simulink model "ObjectDetectLabConditions"  (R2019a)
settings: Solver=FixedStepAuto  StartTime=0.0  StopTime=inf  RelTol=1e-3  EnableMultiTasking=on
undefined symbols (not defined in the file): strel
libraries: embdlinuxlib x5, visionstatistics x1, visiontextngfix x1, visionmorphops x1
settings Model: SimulationMode=external  Creator=Shilpa  LastModifiedBy=Shilpa
settings SolverCC: PositivePriorityOrder=on
settings DataIOCC: ReturnWorkspaceOutputs=off
settings OptimizationCC: PassReuseOutputArgsAs=Individual arguments  MaxStackSize=64
settings DebuggingCC: ParameterTunabilityLossMsg=error  ArithmeticOperatorsInVariantConditions=warning
settings HardwareCC: ProdBitPerPointer=32  ProdBitPerSizeT=32  ProdBitPerPtrDiffT=32  ProdLargestAtomicInteger=Long  ProdLargestAtomicFloat=Double  ProdWordSize=32  ProdHWDeviceType=ARM Compatible->ARM Cortex
settings ModelReferenceCC: UpdateModelReferenceTargets=Force
settings SFSimCC: SimUseLocalCustomCode=off  MATLABDynamicMemAlloc=off
settings RTWCC: SystemTargetFile=ert.tlc  HardwareBoard=Raspberry Pi  TLCOptions="-aInlineSetEventsForThisBaseRateFcn=TLC_FALSE -aSuppressMultiTaskScheduler=TLC_FALSE  -aRateBasedStepFcn=0"  TemplateMakefile=ert_default_tmf  GenerateReport=on  RTWUseLocalCustomCode=off  Toolchain=GNU GCC Raspberry Pi  IncludeHyperlinkInReport=on  LaunchReport=on  GenerateTraceInfo=on  GenerateTraceReport=on  GenerateTraceReportSl=on  GenerateTraceReportSf=on  GenerateTraceReportEml=on
settings CodeAppCC: ForceParamTrailComments=on  IgnoreCustomStorageClasses=off  OperatorAnnotations=on  SimulinkDataObjDesc=on  SFDataObjDesc=on  MATLABFcnDesc=on  InsertBlockDesc=on  StateflowObjectComments=on  MATLABSourceComments=on
settings ERTTargetCC: SupportVariableSizeSignals=on

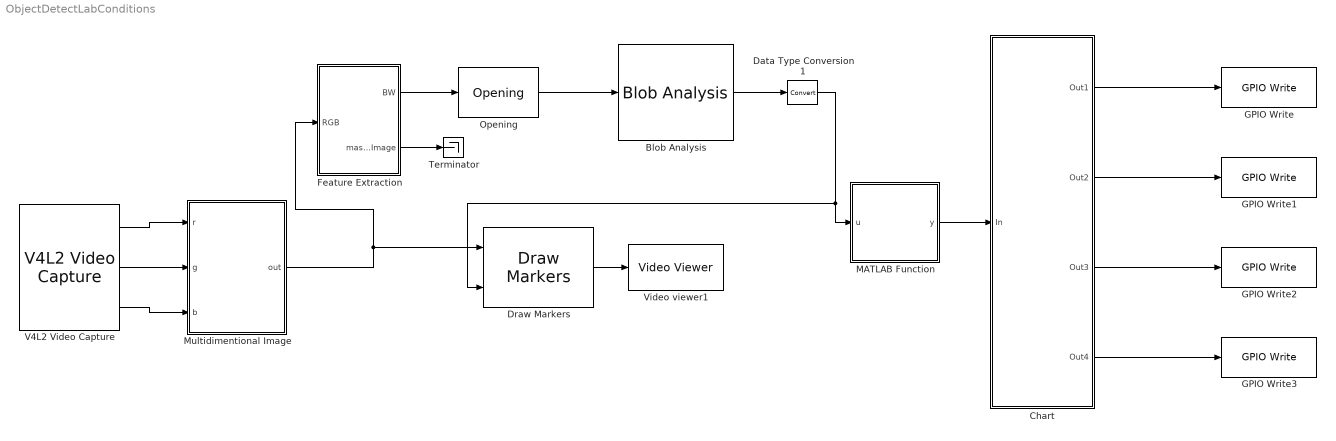
== system ObjectDetectLabConditions ==
  Blob Analysis : visionstatistics/Blob Analysis  Tag=vipblks_row_conv  area=off  centroid=on  bBox=off  majorAxis=off  minorAxis=off  angle=off  eccentricity=off  equivDiameterSq=off  extent=off  perimeter=off  outDT=double  conn=8  isLabel=off  maxBlobs=50  warnIfNumBlobsExceeded=on  isCount=off  useMinArea=off  minArea=0  useMaxArea=off  maxArea=intmax('uint32')  excludeBorderBlob=off  isOutVarDim=off  isFill=on  fillValues=-1  roundingMode=Floor  overflowMode=off  prodOutputMode=Binary point scaling  prodOutputWordLength=32  prodOutputFracLength=16  prodOutputSlope=2^-16  accumMode=Binary point scaling  accumWordLength=32  accumFracLength=0  accumSlope=2^0  outputMode=Binary point scaling  outputWordLength=32  outputFracLength=16  outputSlope=2^-16  memorySlope=2^-16  firstCoeffMode=Binary point scaling  firstCoeffWordLength=16  firstCoeffFracLength=14  firstCoeffSlope=2^-14  secondCoeffMode=Binary point scaling  secondCoeffWordLength=32  secondCoeffFracLength=16  secondCoeffSlope=2^-16
      settings: SourceProductName=Computer Vision Toolbox
  Chart : Stateflow chart  TreatAsAtomicUnit=on
  Data Type Conversion1 : DataTypeConversion
  Draw Markers : visiontextngfix/Draw Markers  shape=X-mark  size=4  fill=off  fillClrSource=Specify via dialog  display=White  intensity=200  color=[200 255 100]  opacity=0.6  viewport=Entire image  antialiasing=off  inType=Obsolete  imagePorts=One multidimensional signal  roundingMode=Floor  overflowMode=off  memoryMode=Specify word length  memoryWordLength=16  memoryFracLength=15  memorySlope=2^-14  prodOutputMode=Binary point scaling  prodOutputWordLength=32  prodOutputFracLength=14  prodOutputSlope=2^-14  accumSlope=2^-14
      settings: SourceProductName=Computer Vision Toolbox  SourceProductBaseCode=VP
  Feature Extraction : MATLAB Function  TreatAsAtomicUnit=on
  GPIO Write : embdlinuxlib/GPIO Write  board=Pi 2 Model B  gpio=23  direction=Output  blockPlatform=Raspberry Pi
      settings: SourceProductName=Simulink Coder Support Package for BeagleBone Blue Hardware  SourceProductBaseCode=SC_BEAGLEBONE_BLUE
  GPIO Write1 : embdlinuxlib/GPIO Write  board=Pi 2 Model B  gpio=24  direction=Output  blockPlatform=Raspberry Pi
      settings: SourceProductName=Simulink Coder Support Package for BeagleBone Blue Hardware  SourceProductBaseCode=SC_BEAGLEBONE_BLUE
  GPIO Write2 : embdlinuxlib/GPIO Write  board=Pi 2 Model B  gpio=27  direction=Output  blockPlatform=Raspberry Pi
      settings: SourceProductName=Simulink Coder Support Package for BeagleBone Blue Hardware  SourceProductBaseCode=SC_BEAGLEBONE_BLUE
  GPIO Write3 : embdlinuxlib/GPIO Write  board=Pi 2 Model B  gpio=22  direction=Output  blockPlatform=Raspberry Pi
      settings: SourceProductName=Simulink Coder Support Package for BeagleBone Blue Hardware  SourceProductBaseCode=SC_BEAGLEBONE_BLUE
  MATLAB Function : MATLAB Function  TreatAsAtomicUnit=on
  Multidimentional Image : MATLAB Function  TreatAsAtomicUnit=on
  Opening : visionmorphops/Opening  nhoodsrc=Specify via dialog  strel=strel('disk',5)
      settings: SourceProductName=Computer Vision Toolbox  SourceProductBaseCode=VP
  Terminator : Terminator
  V4L2 Video Capture : embdlinuxlib/V4L2 Video Capture  m_devName='/dev/video0'  roi=[0, 0, 640, 480]  imSizeSelection=640x480  imSize=[640, 480]  pixelFormat=RGB  pixelOrder=Planar  sampleTime=1/30  simOutput=Colorbars  blockPlatform=Raspberry Pi
      settings: SourceProductName=Simulink Coder Support Package for BeagleBone Blue Hardware  SourceProductBaseCode=SC_BEAGLEBONE_BLUE
  Video viewer1 : VideoViewer  FigPos=[816 654 410 307]
  wires:
  Multidimentional Image/1(out) -> Feature Extraction/1(RGB), Draw Markers/1
  Chart/1(Out1) -> GPIO Write/1
  MATLAB Function/1(y) -> Chart/1(In)
  V4L2 Video Capture/2 -> Multidimentional Image/2(g)
  Feature Extraction/1(BW) -> Opening/1
  Chart/2(Out2) -> GPIO Write1/1
  Chart/4(Out4) -> GPIO Write3/1
  Blob Analysis/1 -> Data Type Conversion1/1
  Chart/3(Out3) -> GPIO Write2/1
  V4L2 Video Capture/3 -> Multidimentional Image/3(b)
  Data Type Conversion1/1 -> MATLAB Function/1(u), Draw Markers/2
  Opening/1 -> Blob Analysis/1
  V4L2 Video Capture/1 -> Multidimentional Image/1(r)
  Feature Extraction/2(maskedRGBImage) -> Terminator/1
  Draw Markers/1 -> Video viewer1/1

== matlab function ObjectDetectLabConditions/Multidimentional Image ==
  data: r input; out output; g input; b input
function out = m_image(r,g,b)
% Converting seperate R,G,B signals into single multidimentional image
out = cat(3,r,g,b);
end

== stateflow chart ObjectDetectLabConditions/Chart ==
  (default) -> (junction 18) : % DC motor
  (junction 18) -> (junction 19) [order 1] : [In(1,2)>360]
  (junction 18) -> (junction 20) [order 2]
  (junction 19) -> (junction 27) : {Out1=1; Out2=0; Out3=1; Out4=0;}
  (junction 20) -> (junction 21) [order 1] : [In(1,2)<120]
  (junction 20) -> (junction 22) [order 2]
  (junction 21) -> (junction 26) : {Out1=0; Out2=1; Out3=0; Out4=1;}
  (junction 22) -> (junction 23) [order 1] : [In(1,1)<150 && (120<In(1,2)<360)]
  (junction 22) -> (junction 29) [order 2]
  (junction 23) -> (junction 25) : {Out1=0; Out2=1; Out3=1; Out4=0;}
  (junction 29) -> (junction 31) [order 1] : [In(1,1)>330 && (120<In(1,2)<360)]
  (junction 29) -> (junction 24) [order 2] : {Out1=0;  Out2=0; Out3=0; Out4=0 ;}
  (junction 31) -> (junction 33) : {Out1=1;Out2=0; Out3=0; Out4=1 ;}
  (junction 33) -> (junction 24)
  (junction 25) -> (junction 33)
  (junction 26) -> (junction 25)
  (junction 27) -> (junction 26)
  (junction 24) -> (junction 28)
  data: In input [1..5]; Out1 output [0..1]; Out2 output [0..1]; Out3 output [0..1]; Out4 output [0..1]

== matlab function ObjectDetectLabConditions/Feature Extraction ==
  data: RGB input; BW output; maskedRGBImage output
function [BW,maskedRGBImage] = createMask(RGB)
%  [BW,MASKEDRGBIMAGE] = createMask(RGB) thresholds image RGB using
%  auto-generated code from the colorThresholder App. The colorspace and
%  minimum/maximum values for each channel of the colorspace were set 
%  and result in a binary mask BW and a composite image maskedRGBImage,
%  which shows the original RGB image values under the mask BW.

% Auto-generated by colorThresholder app on 28-Apr-2017
%------------------------------------------------------


% Convert RGB image to chosen color space
I = rgb2hsv(RGB);

% Define thresholds for channel 1 based on histogram settings
channel1Min = 0.145;
channel1Max = 0.417;

% Define thresholds for channel 2 based on histogram settings
channel2Min = 0.087;
channel2Max = 0.527;

% Define thresholds for channel 3 based on histogram settings
channel3Min = 0.173;
channel3Max = 0.667;

% Create mask based on chosen histogram thresholds
sliderBW = (I(:,:,1) >= channel1Min ) & (I(:,:,1) <= channel1Max) & ...
    (I(:,:,2) >= channel2Min ) & (I(:,:,2) <= channel2Max) & ...
    (I(:,:,3) >= channel3Min ) & (I(:,:,3) <= channel3Max);
BW = sliderBW;

% Initialize output masked image based on input image.
maskedRGBImage = RGB;

% Set background pixels where BW is false to zero.
maskedRGBImage(repmat(~BW,[1 1 3])) = 0;

end

== matlab function ObjectDetectLabConditions/MATLAB Function ==
  data: u input; y output
function y = fcn(u)

y = mean(u);
